simulink model "Model_4"  (R2021b)
settings: Solver=VariableStepAuto  StartTime=0.0  StopTime=10.0  RelTol=1e-3
InitFcn:
  | x_ref = 1; l_ref =0.2; l_ini = 0.7;
  | 
  | %ADRC' s parameter caculation
  | b0 = (ml+mc)/(mc*ml +mc*mt+ml*mt);k_ESO = 15;T_set  = 3;
  | 
  | s_cl = -5.85/T_set;
  | Kp   = s_cl^2;
  | Kd   = -2*s_cl;
  | 
  | s_ESO = k_ESO*s_cl;
  | l1        = -3*s_ESO;
  | l2        = 3*( s_ESO)^2;
  | l3        = -(s_ESO)^3;
  | 
  | %Observer
  | A = [-l1, 1, 0;
  |         -l2, 0, 1;
  |         -l3, 0, 0];
  | B = [0;
  |         b0;
  |         0];
  | L = [l1;
  |        l2;
  |        l3];
  | 
  | b1 = (mt+mc)/(mc*ml +mc*mt+ml*mt);k_ESO1 =90;T_set1  =3;
  | s_cl1 = -5.85/T_set1;
  | Kp1   = s_cl1^2;
  | Kd1   = -2*s_cl1;
  | 
  | s_ESO1 = k_ESO1*s_cl1;
  | l11        = -3*s_ESO1;
  | l21        = 3*( s_ESO1)^2;
  | l31        = -(s_ESO1)^3;
  | 
  | %Observer
  | A1 = [-l11, 1, 0;
  |         -l21, 0, 1;
  |         -l31, 0, 0];
  | B1 = [0;
  |         b1;
  |         0];
  | L1 = [l11;
  |        l21;
  |        l31];
values from neighbouring files (symbols this model uses):
  g = 9.81    [Thong_so_double_pendulum.m]
undefined symbols (not defined in the file or in its folder): data_model41, i, l, mc, o, particle, sigbuilder_block
libraries: neural x166, simulink x5, simulink_extras x5
(part 4 of 4)

== system Model_4/Subsystem5/Radial Basis Network/Layer 2/Delays 1 ==
  "p{2}" : Inport  PortDimensions=153
      mask Display: e = 0.06;c1 = [120 230 180]/255;c2 = ([120 230 180]+0)/(256+128);c3 = ([120 230 180]+128)/(256+128);patch([0 1 1 0],[0 0 1 1],c1);patch([0 1 1 1-e 1-e 0+e],[0 0 1 1-e 0+e 0+e],c2);patch([0 0 1 1-e 0+e 0+e],[0 1 1 1-e 1-e 0+e],c3);plot([0 1 1 0 0],[0 0 1 1 0]);
  mux : Mux  Inputs=1
      mask Display: e = 0.06;c1 = [120 150 230]/255;c2 = ([120 150 230]+0)/383;c3 = ([120 150 230]+128)/383;patch([0 1 1 0],[0 0 1 1],c1);patch([0 1 1 1-e 1-e 0+e],[0 0 1 1-e 0+e 0+e],c2);patch([0 0 1 1-e 0+e 0+e],[0 1 1 1-e 1-e 0+e],c3);plot([0 1 1 0 0],[0 0 1 1 0]);disp('Mux')
  "pd{2,1}" : Outport
      mask Display: e = 0.06;c1 = [120 230 180]/255;c2 = ([120 230 180]+0)/(256+128);c3 = ([120 230 180]+128)/(256+128);patch([0 1 1 0],[0 0 1 1],c1);patch([0 1 1 1-e 1-e 0+e],[0 0 1 1-e 0+e 0+e],c2);patch([0 0 1 1-e 0+e 0+e],[0 1 1 1-e 1-e 0+e],c3);plot([0 1 1 0 0],[0 0 1 1 0]);
  wires:
  "p{2}"/1 -> mux/1
  mux/1 -> "pd{2,1}"/1

== system Model_4/Subsystem5/Radial Basis Network/Layer 2/LW{2,1} ==
  "ad{2,1}" : Inport  PortDimensions=153
      mask Display: e = 0.06;c1 = [120 230 180]/255;c2 = ([120 230 180]+0)/(256+128);c3 = ([120 230 180]+128)/(256+128);patch([0 1 1 0],[0 0 1 1],c1);patch([0 1 1 1-e 1-e 0+e],[0 0 1 1-e 0+e 0+e],c2);patch([0 0 1 1-e 0+e 0+e],[0 1 1 1-e 1-e 0+e],c3);plot([0 1 1 0 0],[0 0 1 1 0]);
  "IW{2,1}(1,:)'" : Constant  Value=[-5184632.5195197947323322296142578125;-20008793.445969425141811370849609375;436989576.98391044139862060546875;503393721.090770065784454345703125;0;0;0;0;0;0;0;0;0;0;0;0;0;0;0;0;0;0;0;0;0;0;0;0;0;0;0;0;0;0;-17113516.9506440460681915283203125;0;0;0;0;-8185425.673346190713346004486083984375;0;0;0;0;14709053.606119669973850250244140625;0;0;0;0;0;0;0;35741729.234374187886714935302734375;0;0;771180404.65598666667938232421875;0;0;0;0;305328746.3394644260406494140625;-1050057378.57425844669342041015625;-1036321333.78514969348907470703125;0;0;0;0;0;0;0;0;0;0;735634015.9430558681488037109375;0;0;0;0;0;0;0;0;0;0;0;0;0;0;0;0;0;-725744720.4771716594696044921875;0;0;0;0;0;0;0;0;0;0;0;0;963503987.23482191562652587890625;0;0;0;0;0;0;0;654528525.5854203701019287109375;0;0;0;0;0;0;0;0;0;0;0;0;1127522526.201610565185546875;0;0;0;0;0;0;0;0;0;0;0;-1588965159.5241525173187255859375;0;0;0;0;0;-660135124.08904922008514404296875;0;0;0;0;0;-436780941.079456031322479248046875;0;0;0]
      mask Display: e = 0.06;c1 = [120 150 230]/255;c2 = ([120 150 230]+0)/383;c3 = ([120 150 230]+128)/383;patch([0 1 1 0],[0 0 1 1],c1);patch([0 1 1 1-e 1-e 0+e],[0 0 1 1-e 0+e 0+e],c2);patch([0 0 1 1-e 0+e 0+e],[0 1 1 1-e 1-e 0+e],c3);plot([0 1 1 0 0],[0 0 1 1 0]);disp('weights');
  "IW{2,1}(2,:)'" : Constant  Value=[-6067249.115095959044992923736572265625;-42417427.302243642508983612060546875;705106361.36008822917938232421875;763664296.7115833759307861328125;0;0;0;0;0;0;0;0;0;0;0;0;0;0;0;0;0;0;0;0;0;0;0;0;0;0;0;0;0;0;-50921722.240085579454898834228515625;0;0;0;0;6622714.44601658545434474945068359375;0;0;0;0;12061934.20341981947422027587890625;0;0;0;0;0;0;0;80654305.1853282153606414794921875;0;0;1262688264.1386871337890625;0;0;0;0;477923137.912937343120574951171875;-1696266297.6033179759979248046875;-1573782889.60526275634765625;0;0;0;0;0;0;0;0;0;0;1120014816.5870258808135986328125;0;0;0;0;0;0;0;0;0;0;0;0;0;0;0;0;0;-1132560889.7355816364288330078125;0;0;0;0;0;0;0;0;0;0;0;0;1559683281.255830287933349609375;0;0;0;0;0;0;0;1016034570.6096017360687255859375;0;0;0;0;0;0;0;0;0;0;0;0;1841697151.355581760406494140625;0;0;0;0;0;0;0;0;0;0;0;-2599663679.627784252166748046875;0;0;0;0;0;-1073182105.8878176212310791015625;0;0;0;0;0;-671231552.57663285732269287109375;0;0;0]
      mask Display: e = 0.06;c1 = [120 150 230]/255;c2 = ([120 150 230]+0)/383;c3 = ([120 150 230]+128)/383;patch([0 1 1 0],[0 0 1 1],c1);patch([0 1 1 1-e 1-e 0+e],[0 0 1 1-e 0+e 0+e],c2);patch([0 0 1 1-e 0+e 0+e],[0 1 1 1-e 1-e 0+e],c3);plot([0 1 1 0 0],[0 0 1 1 0]);disp('weights');
  Mux : Mux  Inputs=2
      mask Display: e = 0.06;c1 = [120 150 230]/255;c2 = ([120 150 230]+0)/383;c3 = ([120 150 230]+128)/383;patch([0 1 1 0],[0 0 1 1],c1);patch([0 1 1 1-e 1-e 0+e],[0 0 1 1-e 0+e 0+e],c2);patch([0 0 1 1-e 0+e 0+e],[0 1 1 1-e 1-e 0+e],c3);plot([0 1 1 0 0],[0 0 1 1 0]);disp('Mux');
  dotprod1 : neural/Weight Functions/dotprod
  dotprod2 : neural/Weight Functions/dotprod
  "lz{2,1}" : Outport
      mask Display: e = 0.06;c1 = [120 230 180]/255;c2 = ([120 230 180]+0)/(256+128);c3 = ([120 230 180]+128)/(256+128);patch([0 1 1 0],[0 0 1 1],c1);patch([0 1 1 1-e 1-e 0+e],[0 0 1 1-e 0+e 0+e],c2);patch([0 0 1 1-e 0+e 0+e],[0 1 1 1-e 1-e 0+e],c3);plot([0 1 1 0 0],[0 0 1 1 0]);
  wires:
  "IW{2,1}(1,:)'"/1 -> dotprod1/1
  "ad{2,1}"/1 -> dotprod1/2, dotprod2/2
  dotprod1/1 -> Mux/1
  "IW{2,1}(2,:)'"/1 -> dotprod2/1
  dotprod2/1 -> Mux/2
  Mux/1 -> "lz{2,1}"/1

== matlab function Model_4/Subsystem5/Subsystem/Crane ==
  data: dx1 output; x2 input; x3 input; x4 input; x5 input; x6 input; Fx input; Fl input; dx2 output; dx3 output; dx4 output; dx5 output; dx6 output; Dp input; mp input
function [dx1,dx2,dx3,dx4,dx5,dx6] = fcn(x2,x3,x4,x5,x6,Fx,Fl,Dp,mp)
 mt =5; mh =2; Dt =20; Dl =50;  g =9.81;

dx1 = x2;
dx2 = (Fx*x3*mh + Fx*x3*mp + Dp*x6*mh*cos(x5) + Dp*x6*mp*cos(x5) - Fl*x3*mp*sin(x5) - x6^2*x3^2*mp^2*sin(x5) ...
+ x2^2*x3^2*mp^2*sin(x5) - Dt*x2*x3*mh - Dt*x2*x3*mp + x2^2*x3^2*mh*mp*sin(x5) + Dl*x4*x3*mp*sin(x5) ...
+ g*x3*mh*mp*cos(x5)*sin(x5))/(x3*(mh*mp + mh*mt + mp*mt - mp^2*cos(x5)^2 - mp^2*sin(x5)^2 + mp^2 - mh*mp*cos(x5)^2));

% d2x = (Fx*l*mh + Fx*l*mp + Dp*d1the*mh*cos(the) + Dp*d1the*mp*cos(the) - Fl*l*mp*sin(the) - d1the^2*l^2*mp^2*sin(the) ...
% + d1x^2*l^2*mp^2*sin(the) - Dt*d1x*l*mh - Dt*d1x*l*mp + d1x^2*l^2*mh*mp*sin(the) + Dl*d1l*l*mp*sin(the) ...
% + g*l*mh*mp*cos(the)*sin(the))/(l*(mh*mp + mh*mt + mp*mt - mp^2*cos(the)^2 - mp^2*sin(the)^2 + mp^2 - mh*mp*cos(the)^2));


dx3 = x4;
dx4 = -(x2^2*x3^2*mp^2*sin(x5)^2 - Fl*x3*mt - x6^2*x3^2*mp^2 - Fl*x3*mp + g*x3*mp^2*cos(x5)^3 + Fx*x3*mp*sin(x5)... 
    + Fl*x3*mp*cos(x5)^2 - x6^2*x3^2*mp*mt - g*x3*mp^2*cos(x5) + Dl*x4*x3*mp + Dl*x4*x3*mt + x6^2*x3^2*mp^2*cos(x5)^2 ...
- Dl*x4*x3*mp*cos(x5)^2 + g*x3*mp^2*cos(x5)*sin(x5)^2 + Dp*x6*mp*cos(x5)*sin(x5) - Dt*x2*x3*mp*sin(x5) ...
    - g*x3*mp*mt*cos(x5))/(x3*(mh*mp + mh*mt + mp*mt - mp^2*cos(x5)^2 - mp^2*sin(x5)^2 + mp^2 - mh*mp*cos(x5)^2));

% d2l = -(d1x^2*l^2*mp^2*sin(the)^2 - Fl*l*mt - d1the^2*l^2*mp^2 - Fl*l*mp + g*l*mp^2*cos(the)^3 + Fx*l*mp*sin(the)... 
%     + Fl*l*mp*cos(the)^2 - d1the^2*l^2*mp*mt - g*l*mp^2*cos(the) + Dl*d1l*l*mp + Dl*d1l*l*mt + d1the^2*l^2*mp^2*cos(the)^2...
% - Dl*d1l*l*mp*cos(the)^2 + g*l*mp^2*cos(the)*sin(the)^2 + Dp*d1the*mp*cos(the)*sin(the) - Dt*d1x*l*mp*sin(the) ...
%     - g*l*mp*mt*cos(the))/(l*(mh*mp + mh*mt + mp*mt - mp^2*cos(the)^2 - mp^2*sin(the)^2 + mp^2 - mh*mp*cos(the)^2));

dx5 = x6;
dx6 = -(Dp*x6*mp^2 - Dp*x6*mp^2*sin(x5)^2 - g*x3*mp^3*sin(x5)^3 + 2*x4*x6*x3*mp^3 + Fx*x3*mp^2*cos(x5) ...
    + Dp*x6*mh*mp + Dp*x6*mh*mt + Dp*x6*mp*mt + g*x3*mp^3*sin(x5) - Dt*x2*x3*mp^2*cos(x5) ...
    - g*x3*mp^3*cos(x5)^2*sin(x5) + g*x3*mh*mp^2*sin(x5) + g*x3*mp^2*mt*sin(x5) - x6^2*x3^2*mp^3*cos(x5)*sin(x5)...
    + x2^2*x3^2*mp^3*cos(x5)*sin(x5) - 2*x4*x6*x3*mp^3*cos(x5)^2 - Fl*x3*mp^2*cos(x5)*sin(x5) ...
    - 2*x4*x6*x3*mp^3*sin(x5)^2 + Fx*x3*mh*mp*cos(x5) + 2*x4*x6*x3*mh*mp^2 + 2*x4*x6*x3*mp^2*mt ...
    + Dl*x4*x3*mp^2*cos(x5)*sin(x5) - 2*x4*x6*x3*mh*mp^2*cos(x5)^2 - Dt*x2*x3*mh*mp*cos(x5) ...
    + g*x3*mh*mp*mt*sin(x5) + 2*x4*x6*x3*mh*mp*mt + x2^2*x3^2*mh*mp^2*cos(x5)*sin(x5))/(x3^2*mp*(mh*mp ...
    + mh*mt + mp*mt - mp^2*cos(x5)^2 - mp^2*sin(x5)^2 + mp^2 - mh*mp*cos(x5)^2));

% d2the = -(Dp*d1the*mp^2 - Dp*d1the*mp^2*sin(the)^2 - g*l*mp^3*sin(the)^3 + 2*d1l*d1the*l*mp^3 + Fx*l*mp^2*cos(the) ...
%     + Dp*d1the*mh*mp + Dp*d1the*mh*mt + Dp*d1the*mp*mt + g*l*mp^3*sin(the) - Dt*d1x*l*mp^2*cos(the) ...
%     - g*l*mp^3*cos(the)^2*sin(the) + g*l*mh*mp^2*sin(the) + g*l*mp^2*mt*sin(the) - d1the^2*l^2*mp^3*cos(the)*sin(the)...
%     + d1x^2*l^2*mp^3*cos(the)*sin(the) - 2*d1l*d1the*l*mp^3*cos(the)^2 - Fl*l*mp^2*cos(the)*sin(the) ...
%     - 2*d1l*d1the*l*mp^3*sin(the)^2 + Fx*l*mh*mp*cos(the) + 2*d1l*d1the*l*mh*mp^2 + 2*d1l*d1the*l*mp^2*mt ...
%     + Dl*d1l*l*mp^2*cos(the)*sin(the) - 2*d1l*d1the*l*mh*mp^2*cos(the)^2 - Dt*d1x*l*mh*mp*cos(the) ...
%     + g*l*mh*mp*mt*sin(the) + 2*d1l*d1the*l*mh*mp*mt + d1x^2*l^2*mh*mp^2*cos(the)*sin(the))/(l^2*mp*(mh*mp ...
%     + mh*mt + mp*mt - mp^2*cos(the)^2 - mp^2*sin(the)^2 + mp^2 - mh*mp*cos(the)^2));

== matlab function Model_4/Subsystem5/ZVD1/MATLAB Function ==
  data: u input; y output
function y = fcn(u)
g = 9.81;
y = pi/sqrt(g/u);

== matlab function Model_4/Subsystem5/ZVD1/MATLAB Function1 ==
  data: u input; y output
function y = fcn(u)
g = 9.81;
y = 2*pi/sqrt(g/u);

== matlab function Model_4/AOF/ZVD1/MATLAB Function ==
  data: u input; y output
function y = fcn(u)
g = 9.81;
y = pi/sqrt(g/u);

== matlab function Model_4/AOF/ZVD1/MATLAB Function1 ==
  data: u input; y output
function y = fcn(u)
g = 9.81;
y = 2*pi/sqrt(g/u);

== matlab function Model_4/Subsystem3/Subsystem/Crane ==
  data: dx1 output; x2 input; x3 input; x4 input; x5 input; x6 input; Fx input; Fl input; dx2 output; dx3 output; dx4 output; dx5 output; dx6 output; mp input; Dp input
function [dx1,dx2,dx3,dx4,dx5,dx6] = fcn(x2,x3,x4,x5,x6,Fx,Fl,mp,Dp)
 mt =5; mh =2; Dt =20; Dl =50;  g =9.81;

dx1 = x2;
dx2 = (Fx*x3*mh + Fx*x3*mp + Dp*x6*mh*cos(x5) + Dp*x6*mp*cos(x5) - Fl*x3*mp*sin(x5) - x6^2*x3^2*mp^2*sin(x5) ...
+ x2^2*x3^2*mp^2*sin(x5) - Dt*x2*x3*mh - Dt*x2*x3*mp + x2^2*x3^2*mh*mp*sin(x5) + Dl*x4*x3*mp*sin(x5) ...
+ g*x3*mh*mp*cos(x5)*sin(x5))/(x3*(mh*mp + mh*mt + mp*mt - mp^2*cos(x5)^2 - mp^2*sin(x5)^2 + mp^2 - mh*mp*cos(x5)^2));

% d2x = (Fx*l*mh + Fx*l*mp + Dp*d1the*mh*cos(the) + Dp*d1the*mp*cos(the) - Fl*l*mp*sin(the) - d1the^2*l^2*mp^2*sin(the) ...
% + d1x^2*l^2*mp^2*sin(the) - Dt*d1x*l*mh - Dt*d1x*l*mp + d1x^2*l^2*mh*mp*sin(the) + Dl*d1l*l*mp*sin(the) ...
% + g*l*mh*mp*cos(the)*sin(the))/(l*(mh*mp + mh*mt + mp*mt - mp^2*cos(the)^2 - mp^2*sin(the)^2 + mp^2 - mh*mp*cos(the)^2));


dx3 = x4;
dx4 = -(x2^2*x3^2*mp^2*sin(x5)^2 - Fl*x3*mt - x6^2*x3^2*mp^2 - Fl*x3*mp + g*x3*mp^2*cos(x5)^3 + Fx*x3*mp*sin(x5)... 
    + Fl*x3*mp*cos(x5)^2 - x6^2*x3^2*mp*mt - g*x3*mp^2*cos(x5) + Dl*x4*x3*mp + Dl*x4*x3*mt + x6^2*x3^2*mp^2*cos(x5)^2 ...
- Dl*x4*x3*mp*cos(x5)^2 + g*x3*mp^2*cos(x5)*sin(x5)^2 + Dp*x6*mp*cos(x5)*sin(x5) - Dt*x2*x3*mp*sin(x5) ...
    - g*x3*mp*mt*cos(x5))/(x3*(mh*mp + mh*mt + mp*mt - mp^2*cos(x5)^2 - mp^2*sin(x5)^2 + mp^2 - mh*mp*cos(x5)^2));

% d2l = -(d1x^2*l^2*mp^2*sin(the)^2 - Fl*l*mt - d1the^2*l^2*mp^2 - Fl*l*mp + g*l*mp^2*cos(the)^3 + Fx*l*mp*sin(the)... 
%     + Fl*l*mp*cos(the)^2 - d1the^2*l^2*mp*mt - g*l*mp^2*cos(the) + Dl*d1l*l*mp + Dl*d1l*l*mt + d1the^2*l^2*mp^2*cos(the)^2...
% - Dl*d1l*l*mp*cos(the)^2 + g*l*mp^2*cos(the)*sin(the)^2 + Dp*d1the*mp*cos(the)*sin(the) - Dt*d1x*l*mp*sin(the) ...
%     - g*l*mp*mt*cos(the))/(l*(mh*mp + mh*mt + mp*mt - mp^2*cos(the)^2 - mp^2*sin(the)^2 + mp^2 - mh*mp*cos(the)^2));

dx5 = x6;
dx6 = -(Dp*x6*mp^2 - Dp*x6*mp^2*sin(x5)^2 - g*x3*mp^3*sin(x5)^3 + 2*x4*x6*x3*mp^3 + Fx*x3*mp^2*cos(x5) ...
    + Dp*x6*mh*mp + Dp*x6*mh*mt + Dp*x6*mp*mt + g*x3*mp^3*sin(x5) - Dt*x2*x3*mp^2*cos(x5) ...
    - g*x3*mp^3*cos(x5)^2*sin(x5) + g*x3*mh*mp^2*sin(x5) + g*x3*mp^2*mt*sin(x5) - x6^2*x3^2*mp^3*cos(x5)*sin(x5)...
    + x2^2*x3^2*mp^3*cos(x5)*sin(x5) - 2*x4*x6*x3*mp^3*cos(x5)^2 - Fl*x3*mp^2*cos(x5)*sin(x5) ...
    - 2*x4*x6*x3*mp^3*sin(x5)^2 + Fx*x3*mh*mp*cos(x5) + 2*x4*x6*x3*mh*mp^2 + 2*x4*x6*x3*mp^2*mt ...
    + Dl*x4*x3*mp^2*cos(x5)*sin(x5) - 2*x4*x6*x3*mh*mp^2*cos(x5)^2 - Dt*x2*x3*mh*mp*cos(x5) ...
    + g*x3*mh*mp*mt*sin(x5) + 2*x4*x6*x3*mh*mp*mt + x2^2*x3^2*mh*mp^2*cos(x5)*sin(x5))/(x3^2*mp*(mh*mp ...
    + mh*mt + mp*mt - mp^2*cos(x5)^2 - mp^2*sin(x5)^2 + mp^2 - mh*mp*cos(x5)^2));

% d2the = -(Dp*d1the*mp^2 - Dp*d1the*mp^2*sin(the)^2 - g*l*mp^3*sin(the)^3 + 2*d1l*d1the*l*mp^3 + Fx*l*mp^2*cos(the) ...
%     + Dp*d1the*mh*mp + Dp*d1the*mh*mt + Dp*d1the*mp*mt + g*l*mp^3*sin(the) - Dt*d1x*l*mp^2*cos(the) ...
%     - g*l*mp^3*cos(the)^2*sin(the) + g*l*mh*mp^2*sin(the) + g*l*mp^2*mt*sin(the) - d1the^2*l^2*mp^3*cos(the)*sin(the)...
%     + d1x^2*l^2*mp^3*cos(the)*sin(the) - 2*d1l*d1the*l*mp^3*cos(the)^2 - Fl*l*mp^2*cos(the)*sin(the) ...
%     - 2*d1l*d1the*l*mp^3*sin(the)^2 + Fx*l*mh*mp*cos(the) + 2*d1l*d1the*l*mh*mp^2 + 2*d1l*d1the*l*mp^2*mt ...
%     + Dl*d1l*l*mp^2*cos(the)*sin(the) - 2*d1l*d1the*l*mh*mp^2*cos(the)^2 - Dt*d1x*l*mh*mp*cos(the) ...
%     + g*l*mh*mp*mt*sin(the) + 2*d1l*d1the*l*mh*mp*mt + d1x^2*l^2*mh*mp^2*cos(the)*sin(the))/(l^2*mp*(mh*mp ...
%     + mh*mt + mp*mt - mp^2*cos(the)^2 - mp^2*sin(the)^2 + mp^2 - mh*mp*cos(the)^2));

== matlab function Model_4/AOL/ZVD1/MATLAB Function ==
  data: u input; y output
function y = fcn(u)
g = 9.81;
y = pi/sqrt(g/u);

== matlab function Model_4/AOL/ZVD1/MATLAB Function1 ==
  data: u input; y output
function y = fcn(u)
g = 9.81;
y = 2*pi/sqrt(g/u);

== matlab function Model_4/Subsystem3/ZVD1/MATLAB Function ==
  data: u input; y output
function y = fcn(u)
g = 9.81;
y = pi/sqrt(g/u);

== matlab function Model_4/Subsystem3/ZVD1/MATLAB Function1 ==
  data: u input; y output
function y = fcn(u)
g = 9.81;
y = 2*pi/sqrt(g/u);

== matlab function Model_4/Subsystem1/Crane ==
  data: x1 input; dx1 output; x2 input; x3 input; x4 input; x5 input; x6 input; ut input; ul input; dx2 output; dx3 output; dx4 output; dx5 output; dx6 output
function [dx1,dx2,dx3,dx4,dx5,dx6] = fcn(x1,x2,x3,x4,x5,x6,ut,ul)
mc = 0.85; mt =5; ml =2; bt =20; br =50; g =9.81;

dx1 = x2;
dx2 = -(bt*x2 *mc - ml*ut - mc*ul*sin(x5) - mc*ut + bt*x2 *ml ...
- x6^2*x3*mc^2*sin(x5) + br*x4*mc*sin(x5) + x6^2*x3*mc*ml*sin(x5) ...
+ g*mc*ml*cos(x5)*sin(x5))/(mc*ml + mc*mt + ml*mt - mc^2*cos(x5)^2 ...
- mc^2*sin(x5)^2 + mc^2 - mc*ml*cos(x5)^2);
% -(bt*d1x*mc - ml*ut - mc*ul*sin(the) - mc*ut + bt*d1x*ml 
% - d1the^2*l*mc^2*sin(the) + br*d1l*mc*sin(the) + d1the^2*l*mc*ml*sin(the) 
% + g*mc*ml*cos(the)*sin(the))/(mc*ml + mc*mt + ml*mt - mc^2*cos(the)^2 
% - mc^2*sin(the)^2 + mc^2 - mc*ml*cos(the)^2)

dx3 = x4;
dx4 = (mc*ul + mt*ul + mc*ut*sin(x5) + 2*x6^2*x3*mc^2 + g*mc^2*cos(x5) ...
- mc*ul*cos(x5)^2 - br*x4*mc - br*x4*mt - g*mc^2*cos(x5)^3 + 2*x6^2*x3*mc*mt ...
+ g*mc*mt*cos(x5) - bt*x2 *mc*sin(x5) - 2*x6^2*x3*mc^2*cos(x5)^2  ...
- x6^2*x3*mc^2*sin(x5)^2 - g*mc^2*cos(x5)*sin(x5)^2 ...
+ br*x4*mc*cos(x5)^2)/(mc*ml + mc*mt + ml*mt - mc^2*cos(x5)^2 ...
- mc^2*sin(x5)^2 + mc^2 - mc*ml*cos(x5)^2);
% (mc*ul + mt*ul + mc*ut*sin(the) + 2*d1the^2*l*mc^2 + g*mc^2*cos(the)
% - mc*ul*cos(the)^2 - br*d1l*mc - br*d1l*mt - g*mc^2*cos(the)^3 + 2*d1the^2*l*mc*mt 
% + g*mc*mt*cos(the) - bt*d1x*mc*sin(the) - 2*d1the^2*l*mc^2*cos(the)^2 
% - d1the^2*l*mc^2*sin(the)^2 - g*mc^2*cos(the)*sin(the)^2 
% + br*d1l*mc*cos(the)^2)/(mc*ml + mc*mt + ml*mt - mc^2*cos(the)^2 
% - mc^2*sin(the)^2 + mc^2 - mc*ml*cos(the)^2)

dx5 = x6;
dx6 = -(g*mc^2*sin(x5) - ml*ut*cos(x5) - mc*ut*cos(x5) - g*mc^2*sin(x5)^3 ...
+ 2*x4*x6*mc^2 - mc*ul*cos(x5)*sin(x5) + 2*x4*x6*mc*ml ...
+ 2*x4*x6*mc*mt + 2*x4*x6*ml*mt - 2*x4*x6*mc^2*cos(x5)^2 ...
- 2*x4*x6*mc^2*sin(x5)^2 + bt*x2 *mc*cos(x5) + bt*x2 *ml*cos(x5)...
+ g*mc*ml*sin(x5) + g*mc*mt*sin(x5) + g*ml*mt*sin(x5) ...
- g*mc^2*cos(x5)^2*sin(x5) - x6^2*x3*mc^2*cos(x5)*sin(x5) ...
- 2*x4*x6*mc*ml*cos(x5)^2 + br*x4*mc*cos(x5)*sin(x5) ...
+ x6^2*x3*mc*ml*cos(x5)*sin(x5))/(x3*(mc*ml + mc*mt + ml*mt ...
- mc^2*cos(x5)^2 - mc^2*sin(x5)^2 + mc^2 - mc*ml*cos(x5)^2));
% -(g*mc^2*sin(the) - ml*ut*cos(the) - mc*ut*cos(the) - g*mc^2*sin(the)^3 
% + 2*d1l*d1the*mc^2 - mc*ul*cos(the)*sin(the) + 2*d1l*d1the*mc*ml 
% + 2*d1l*d1the*mc*mt + 2*d1l*d1the*ml*mt - 2*d1l*d1the*mc^2*cos(the)^2 
% - 2*d1l*d1the*mc^2*sin(the)^2 + bt*d1x*mc*cos(the) + bt*d1x*ml*cos(the) 
% + g*mc*ml*sin(the) + g*mc*mt*sin(the) + g*ml*mt*sin(the) 
% - g*mc^2*cos(the)^2*sin(the) - d1the^2*l*mc^2*cos(the)*sin(the) 
% - 2*d1l*d1the*mc*ml*cos(the)^2 + br*d1l*mc*cos(the)*sin(the) 
% + d1the^2*l*mc*ml*cos(the)*sin(the))/(l*(mc*ml + mc*mt + ml*mt 
% - mc^2*cos(the)^2 - mc^2*sin(the)^2 + mc^2 - mc*ml*cos(the)^2))

== matlab function Model_4/Subsystem2/Subsystem/Crane ==
  data: dx1 output; x2 input; x3 input; x4 input; x5 input; x6 input; ut input; ul input; dx2 output; dx3 output; dx4 output; dx5 output; dx6 output; Dt input; mc input
function [dx1,dx2,dx3,dx4,dx5,dx6] = fcn(x2,x3,x4,x5,x6,ut,ul,Dt,mc)
 mt =5; ml =2; bt =20; br =50;  g =9.81;

dx1 = x2;
dx2= -(bt*x2*mc - ml*ut - mc*ul*sin(x5) - mc*ut + bt*x2*ml - x6^2*x3*mc^2*sin(x5) + br*x4*mc*sin(x5) + Dt*x6*mc^2*cos(x5) + x6^2*x3*mc*ml*sin(x5) + g*mc*ml*cos(x5)*sin(x5) + Dt*x6*mc*ml*cos(x5))/(mc*ml + mc*mt + ml*mt - mc^2*cos(x5)^2 - mc^2*sin(x5)^2 + mc^2 - mc*ml*cos(x5)^2);
 
dx3 = x4;
dx4 = -(mc*ul*cos(x5)^2 - mt*ul - mc*ut*sin(x5) - 2*x6^2*x3*mc^2 - g*mc^2*cos(x5) - mc*ul + br*x4*mc + br*x4*mt + g*mc^2*cos(x5)^3 - 2*x6^2*x3*mc*mt - g*mc*mt*cos(x5) + bt*x2*mc*sin(x5) + 2*x6^2*x3*mc^2*cos(x5)^2 + x6^2*x3*mc^2*sin(x5)^2 + g*mc^2*cos(x5)*sin(x5)^2 - br*x4*mc*cos(x5)^2 + Dt*x6*mc^2*cos(x5)*sin(x5))/(mc*ml + mc*mt + ml*mt - mc^2*cos(x5)^2 - mc^2*sin(x5)^2 + mc^2 - mc*ml*cos(x5)^2);
dx5 = x6;
dx6 = -(g*mc^2*sin(x5) - ml*ut*cos(x5) - mc*ut*cos(x5) + Dt*x6*mc^2 - g*mc^2*sin(x5)^3 + 2*x4*x6*mc^2 - mc*ul*cos(x5)*sin(x5) + 2*x4*x6*mc*ml + 2*x4*x6*mc*mt + 2*x4*x6*ml*mt - Dt*x6*mc^2*sin(x5)^2 - 2*x4*x6*mc^2*cos(x5)^2 - 2*x4*x6*mc^2*sin(x5)^2 + bt*x2*mc*cos(x5) + bt*x2*ml*cos(x5) + g*mc*ml*sin(x5) + g*mc*mt*sin(x5) + g*ml*mt*sin(x5) - g*mc^2*cos(x5)^2*sin(x5) + Dt*x6*mc*ml + Dt*x6*mc*mt + Dt*x6*ml*mt - x6^2*x3*mc^2*cos(x5)*sin(x5) - 2*x4*x6*mc*ml*cos(x5)^2 + br*x4*mc*cos(x5)*sin(x5) + x6^2*x3*mc*ml*cos(x5)*sin(x5))/(x3*(mc*ml + mc*mt + ml*mt - mc^2*cos(x5)^2 - mc^2*sin(x5)^2 + mc^2 - mc*ml*cos(x5)^2));

== matlab function Model_4/AOF/Subsystem2/Crane ==
  data: dx1 output; x2 input; x3 input; x4 input; x5 input; x6 input; ut input; ul input; dx2 output; dx3 output; dx4 output; dx5 output; dx6 output; Dt input; mc input
function [dx1,dx2,dx3,dx4,dx5,dx6] = fcn(x2,x3,x4,x5,x6,ut,ul,Dt,mc)
 mt =5; ml =2; bt =20; br =50;  g =9.81;

dx1 = x2;
dx2= -(bt*x2*mc - ml*ut - mc*ul*sin(x5) - mc*ut + bt*x2*ml - x6^2*x3*mc^2*sin(x5) + br*x4*mc*sin(x5) + Dt*x6*mc^2*cos(x5) ...
    + x6^2*x3*mc*ml*sin(x5) + g*mc*ml*cos(x5)*sin(x5) + Dt*x6*mc*ml*cos(x5))/(mc*ml + mc*mt + ml*mt - mc^2*cos(x5)^2 - mc^2*sin(x5)^2 + mc^2 - mc*ml*cos(x5)^2);
 
dx3 = x4;
dx4 = -(mc*ul*cos(x5)^2 - mt*ul - mc*ut*sin(x5) - 2*x6^2*x3*mc^2 - g*mc^2*cos(x5) - mc*ul + br*x4*mc + br*x4*mt + g*mc^2*cos(x5)^3 - 2*x6^2*x3*mc*mt - g*mc*mt*cos(x5) ...
    + bt*x2*mc*sin(x5) + 2*x6^2*x3*mc^2*cos(x5)^2 + x6^2*x3*mc^2*sin(x5)^2 + g*mc^2*cos(x5)*sin(x5)^2 - br*x4*mc*cos(x5)^2 ...
    + Dt*x6*mc^2*cos(x5)*sin(x5))/(mc*ml + mc*mt + ml*mt - mc^2*cos(x5)^2 - mc^2*sin(x5)^2 + mc^2 - mc*ml*cos(x5)^2);
dx5 = x6;
dx6 = -(g*mc^2*sin(x5) - ml*ut*cos(x5) - mc*ut*cos(x5) + Dt*x6*mc^2 - g*mc^2*sin(x5)^3 + 2*x4*x6*mc^2 - mc*ul*cos(x5)*sin(x5) + 2*x4*x6*mc*ml ...
    + 2*x4*x6*mc*mt + 2*x4*x6*ml*mt - Dt*x6*mc^2*sin(x5)^2 - 2*x4*x6*mc^2*cos(x5)^2 - 2*x4*x6*mc^2*sin(x5)^2 + bt*x2*mc*cos(x5) + bt*x2*ml*cos(x5) ...
    + g*mc*ml*sin(x5) + g*mc*mt*sin(x5) + g*ml*mt*sin(x5) - g*mc^2*cos(x5)^2*sin(x5) + Dt*x6*mc*ml + Dt*x6*mc*mt + Dt*x6*ml*mt - x6^2*x3*mc^2*cos(x5)*sin(x5) ...
    - 2*x4*x6*mc*ml*cos(x5)^2 + br*x4*mc*cos(x5)*sin(x5) + x6^2*x3*mc*ml*cos(x5)*sin(x5))/(x3*(mc*ml + mc*mt + ml*mt - mc^2*cos(x5)^2 - mc^2*sin(x5)^2 + mc^2 - mc*ml*cos(x5)^2));

== matlab function Model_4/AOL/Subsystem/Crane ==
  data: dx1 output; x2 input; x3 input; x4 input; x5 input; x6 input; ut input; ul input; dx2 output; dx3 output; dx4 output; dx5 output; dx6 output; Dt input; mc input
function [dx1,dx2,dx3,dx4,dx5,dx6] = fcn(x2,x3,x4,x5,x6,ut,ul,Dt,mc)
 mt =5; ml =2; bt =20; br =50;  g =9.81;

dx1 = x2;
dx2= -(bt*x2*mc - ml*ut - mc*ul*sin(x5) - mc*ut + bt*x2*ml - x6^2*x3*mc^2*sin(x5) + br*x4*mc*sin(x5) + Dt*x6*mc^2*cos(x5) + x6^2*x3*mc*ml*sin(x5) + g*mc*ml*cos(x5)*sin(x5) + Dt*x6*mc*ml*cos(x5))/(mc*ml + mc*mt + ml*mt - mc^2*cos(x5)^2 - mc^2*sin(x5)^2 + mc^2 - mc*ml*cos(x5)^2);
 
dx3 = x4;
dx4 = -(mc*ul*cos(x5)^2 - mt*ul - mc*ut*sin(x5) - 2*x6^2*x3*mc^2 - g*mc^2*cos(x5) - mc*ul + br*x4*mc + br*x4*mt + g*mc^2*cos(x5)^3 - 2*x6^2*x3*mc*mt - g*mc*mt*cos(x5) + bt*x2*mc*sin(x5) + 2*x6^2*x3*mc^2*cos(x5)^2 + x6^2*x3*mc^2*sin(x5)^2 + g*mc^2*cos(x5)*sin(x5)^2 - br*x4*mc*cos(x5)^2 + Dt*x6*mc^2*cos(x5)*sin(x5))/(mc*ml + mc*mt + ml*mt - mc^2*cos(x5)^2 - mc^2*sin(x5)^2 + mc^2 - mc*ml*cos(x5)^2);
dx5 = x6;
dx6 = -(g*mc^2*sin(x5) - ml*ut*cos(x5) - mc*ut*cos(x5) + Dt*x6*mc^2 - g*mc^2*sin(x5)^3 + 2*x4*x6*mc^2 - mc*ul*cos(x5)*sin(x5) + 2*x4*x6*mc*ml + 2*x4*x6*mc*mt + 2*x4*x6*ml*mt - Dt*x6*mc^2*sin(x5)^2 - 2*x4*x6*mc^2*cos(x5)^2 - 2*x4*x6*mc^2*sin(x5)^2 + bt*x2*mc*cos(x5) + bt*x2*ml*cos(x5) + g*mc*ml*sin(x5) + g*mc*mt*sin(x5) + g*ml*mt*sin(x5) - g*mc^2*cos(x5)^2*sin(x5) + Dt*x6*mc*ml + Dt*x6*mc*mt + Dt*x6*ml*mt - x6^2*x3*mc^2*cos(x5)*sin(x5) - 2*x4*x6*mc*ml*cos(x5)^2 + br*x4*mc*cos(x5)*sin(x5) + x6^2*x3*mc*ml*cos(x5)*sin(x5))/(x3*(mc*ml + mc*mt + ml*mt - mc^2*cos(x5)^2 - mc^2*sin(x5)^2 + mc^2 - mc*ml*cos(x5)^2));
